simulink model "model"  (R2020b)
settings: Solver=VariableStepAuto  StartTime=0.0  StopTime=10.0  RelTol=1e-3
settings Model: Creator=Lenovo  LastModifiedBy=Lenovo

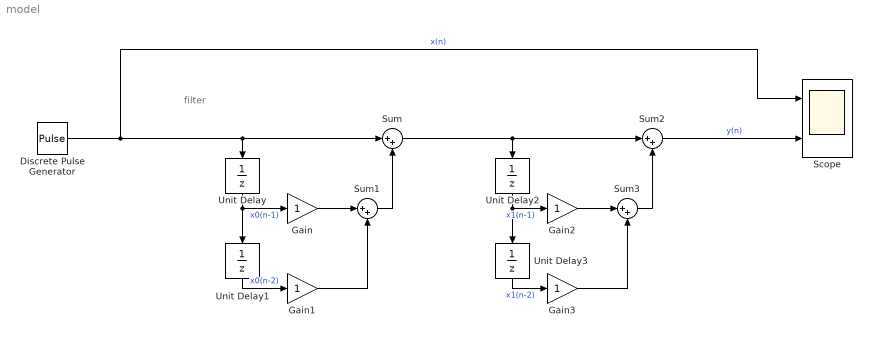
== system model ==
  note: filter
  Discrete Pulse Generator : DiscretePulseGenerator  Period=10  PulseWidth=5
  Gain{,1..3} (4 alike) : Gain
  Scope : Scope  NumInputPorts=2
  Sum{,1..3} (4 alike) : Sum  Inputs=|++
  Unit Delay{,1..3} (4 alike) : UnitDelay  SampleTime=-1  HasFrameUpgradeWarning=on
  wires:
  Discrete Pulse Generator/1 -> Scope/1, Sum/1, Unit Delay/1  "x(n)"
  Unit Delay/1 -> Gain/1, Unit Delay1/1  "x0(n-1)"
  Gain/1 -> Sum1/1
  Unit Delay1/1 -> Gain1/1  "x0(n-2)"
  Gain1/1 -> Sum1/2
  Sum1/1 -> Sum/2
  Unit Delay3/1 -> Gain3/1  "x1(n-2)"
  Unit Delay2/1 -> Gain2/1, Unit Delay3/1  "x1(n-1)"
  Gain2/1 -> Sum3/1
  Gain3/1 -> Sum3/2
  Sum3/1 -> Sum2/2
  Sum/1 -> Unit Delay2/1, Sum2/1
  Sum2/1 -> Scope/2  "y(n)"
